simulink model "kinematic_model_pid"  (R2017a)
settings: Solver=ode45  StartTime=0.0  StopTime=5  RelTol=1e-3  EnableMultiTasking=on
InitFcn:
  | S = 1
  | P = 1
  | I = 1
  | D = 1
values from neighbouring files (symbols this model uses):
  Brot = 0    [param_2224.m]
  Bwheel = 0    [param_2224.m]
  Dist_wheels = 0.12    [param_2224.m]
  Jrot = 2.7e-7    (= 2.7e-07)    [param_2224.m]
  Jwheel = 4.013e-6    (= 4.013e-06)    [param_2224.m]
  Ke = 1.115e-3*60/(2*pi)    (= 0.0106474656928)    [param_2224.m]
  Km = 11.12e-3    (= 0.01112)    [param_2224.m]
  L = 130e-6    (= 0.00013)    [param_2224.m]
  n = 8    [param_2224.m]
  R = 8.71    [param_2224.m]
  rads2mps = Rwheel    (= 0.0325)    [param_2224.m]
  rads2rpm = 60/(2*pi)    (= 9.54929658551)    [param_2224.m]
  ro = 0.9    [param_2224.m]
libraries: simulink x11
settings Model: Creator=void  LastModifiedBy=johne
settings DataIOCC: LimitDataPoints=on  SaveFormat=Array  SignalLoggingSaveFormat=ModelDataLogs
settings OptimizationCC: ExpressionDepthLimit=2147483647  InitFltsAndDblsToZero=on  LifeSpan=inf
settings DebuggingCC: SaveWithParameterizedLinksMsg=none  UnderspecifiedInitializationDetection=Classic  MergeDetectMultiDrivingBlocksExec=none  SignalResolutionControl=TryResolveAllWithWarning  SolverPrmCheckMsg=warning  MultiTaskDSMMsg=warning  MultiTaskCondExecSysMsg=none  FcnCallInpInsideContextMsg=warning  StateNameClashWarn=warning  SFUnexpectedBacktrackingDiag=warning  SFNoUnconditionalDefaultTransitionDiag=warning  SFExecutionAtInitializationDiag=none
settings HardwareCC: ProdBitPerPointer=32  ProdBitPerSizeT=32  ProdBitPerPtrDiffT=32  ProdLargestAtomicFloat=None  ProdIntDivRoundTo=Undefined  ProdEndianess=Unspecified  ProdWordSize=32  ProdHWDeviceType=32-bit Generic
settings ModelReferenceCC: PropagateSignalLabelsOutOfModel=off
settings GRTTargetCC: TargetFcnLib=ansi_tfl_tmw.mat  TargetLangStandard=C89/C90 (ANSI)  GeneratePreprocessorConditionals=Disable all  CombineOutputUpdateFcns=off  GRTInterface=on
settings ConfigComp: CovMetricSettings=dw  CovHtmlReporting=on  CovSaveCumulativeToWorkspaceVar=on  CovSaveSingleToWorkspaceVar=on  CovExternalEMLEnable=off

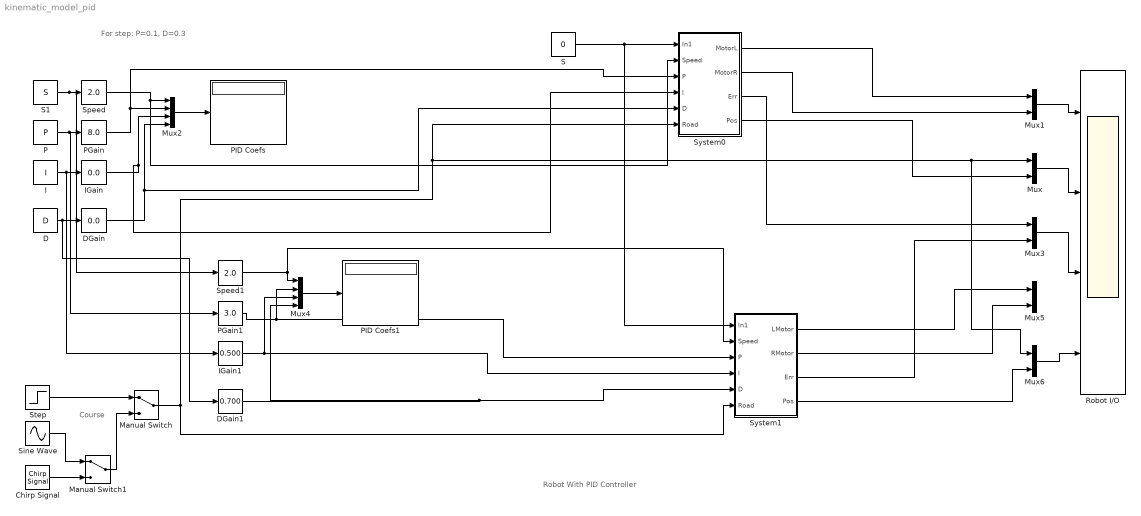
== system kinematic_model_pid ==
  note: For step: P=0.1, D=0.3
  note: Course
  note: Robot With PID Controller
  Chirp Signal : simulink/Sources/Chirp Signal  f1=0.1  T=100  f2=1
  D : Constant  Value=D
  DGain : simulink/Math Operations/Slider Gain  gain=0.0  low=0  high=1
  DGain1 : simulink/Math Operations/Slider Gain  gain=0.700  low=0  high=1
  I : Constant  Value=I
  IGain : simulink/Math Operations/Slider Gain  gain=0.0  low=0  high=1
  IGain1 : simulink/Math Operations/Slider Gain  gain=0.500  low=0  high=1
  Manual Switch : ManualSwitch
  Manual Switch1 : ManualSwitch
  Mux{,1,3,5..6} (5 alike) : Mux  Inputs=2
  Mux2 : Mux
  Mux4 : Mux
  P : Constant  Value=P
  PGain : simulink/Math Operations/Slider Gain  gain=8.0  low=0  high=10
  PGain1 : simulink/Math Operations/Slider Gain  gain=3.0  low=0  high=10
  PID Coefs : Display
  PID Coefs1 : Display
  Robot I/O : Scope  NumInputPorts=4
  S : Constant  Value=0
  S1 : Constant  Value=S
  Sine Wave : Sin  Amplitude=.4  Frequency=2  SampleTime=0
  Speed : simulink/Math Operations/Slider Gain  gain=2.0  low=0  high=10
  Speed1 : simulink/Math Operations/Slider Gain  gain=2.0  low=0  high=10
  Step : Step  After=.5  SampleTime=0
  System0 : Subsystem
  System1 : Subsystem
  wires:
  Speed/1 -> System0/2(Speed), Mux2/1
  Step/1 -> Manual Switch/1
  Manual Switch/1 -> System1/6(Road), System0/6(Road), Mux6/1, Mux/1
  Mux/1 -> Robot I/O/2
  Mux1/1 -> Robot I/O/1
  P/1 -> PGain1/1, PGain/1
  Mux2/1 -> PID Coefs/1
  I/1 -> IGain1/1, IGain/1
  D/1 -> DGain1/1, DGain/1
  Chirp Signal/1 -> Manual Switch1/2
  Manual Switch1/1 -> Manual Switch/2
  Sine Wave/1 -> Manual Switch1/1
  S1/1 -> Speed1/1, Speed/1
  PGain/1 -> System0/3(P), Mux2/2
  IGain/1 -> System0/4(I), Mux2/3
  DGain/1 -> System0/5(D), Mux2/4
  System0/1(MotorL) -> Mux1/1
  System0/2(MotorR) -> Mux1/2
  System0/4(Pos) -> Mux/2
  System0/3(Err) -> Mux3/1
  Mux3/1 -> Robot I/O/3
  System1/3(Err) -> Mux3/2
  Speed1/1 -> System1/2(Speed), Mux4/1
  Mux4/1 -> PID Coefs1/1
  PGain1/1 -> System1/3(P), Mux4/2
  IGain1/1 -> System1/4(I), Mux4/3
  DGain1/1 -> System1/5(D), Mux4/4
  Mux6/1 -> Robot I/O/4
  System1/1(LMotor) -> Mux5/1
  System1/2(RMotor) -> Mux5/2
  System1/4(Pos) -> Mux6/2
  S/1 -> System1/1(In1), System0/1(In1)

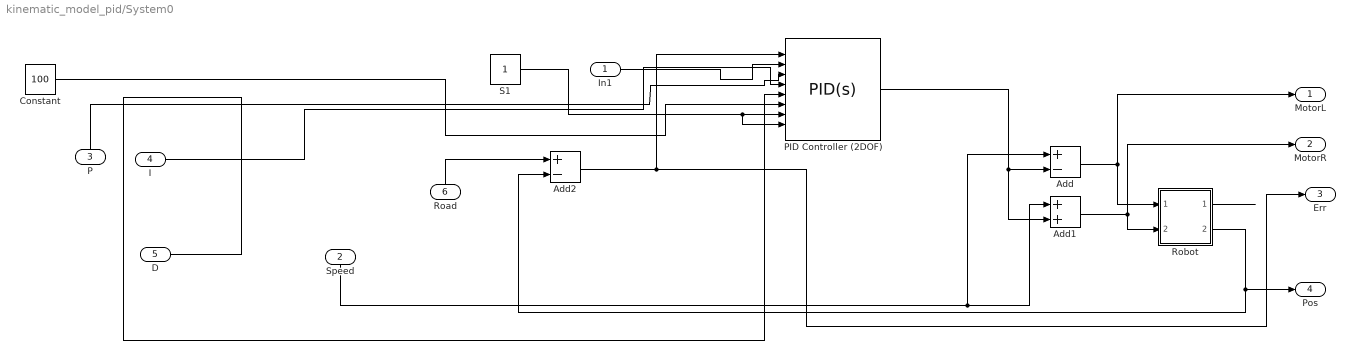
== system kinematic_model_pid/System0 ==
  In1 : Inport
  Speed : Inport  Port=2
  P : Inport  Port=3
  I : Inport  Port=4
  D : Inport  Port=5
  Road : Inport  Port=6
  Add : Sum  Inputs=+-
  Add1 : Sum
  Add2 : Sum  Inputs=+-
  Constant : Constant  Value=100
  PID Controller (2DOF) : simulink/Continuous/PID Controller (2DOF)  Controller=PID  TimeDomain=Continuous-time  SampleTime=-1  IntegratorMethod=Forward Euler  FilterMethod=Forward Euler  Form=Parallel  UseFilter=on  ControllerParametersSource=external  P=1  I=1  D=0  N=100  b=1  c=1  InitialConditionSource=internal  InitialConditionForIntegrator=0  InitialConditionForFilter=0  ExternalReset=none  LimitOutput=off  UpperSaturationLimit=inf  LowerSaturationLimit=-inf  LinearizeAsGain=on  AntiWindupMode=none  Kb=1  TrackingMode=off  Kt=1  PParamMin=[]  PParamMax=[]  IParamMin=[]  IParamMax=[]  DParamMin=[]  DParamMax=[]  NParamMin=[]  NParamMax=[]  bParamMin=[]  bParamMax=[]  cParamMin=[]  cParamMax=[]  KbParamMin=[]  KbParamMax=[]  KtParamMin=[]  KtParamMax=[]  POutMin=[]  POutMax=[]  IOutMin=[]  IOutMax=[]  DOutMin=[]  DOutMax=[]  NOutMin=[]  NOutMax=[]  bOutMin=[]  bOutMax=[]  cOutMin=[]  cOutMax=[]  KbOutMin=[]  KbOutMax=[]  KtOutMin=[]  KtOutMax=[]  IntegratorOutMin=[]  IntegratorOutMax=[]  FilterOutMin=[]  FilterOutMax=[]  SumOutMin=[]  SumOutMax=[]  Sum1OutMin=[]  Sum1OutMax=[]  Sum2OutMin=[]  Sum2OutMax=[]  Sum3OutMin=[]  Sum3OutMax=[]  SumI1OutMin=[]  SumI1OutMax=[]  SumI2OutMin=[]  SumI2OutMax=[]  SumI3OutMin=[]  SumI3OutMax=[]  SumDOutMin=[]  SumDOutMax=[]  SaturationOutMin=[]  SaturationOutMax=[]  IntegratorContinuousStateAttributes=''  IntegratorStateMustResolveToSignalObject=off  IntegratorRTWStateStorageClass=Auto  FilterContinuousStateAttributes=''  FilterStateMustResolveToSignalObject=off  FilterRTWStateStorageClass=Auto  DifferentiatorICPrevScaledInput=0  DifferentiatorOutMin=[]  DifferentiatorOutMax=[]  InitialConditionSetting=State (most efficient)
  Robot : Subsystem
  S1 : Constant
  MotorL : Outport
  MotorR : Outport  Port=2
  Err : Outport  Port=3
  Pos : Outport  Port=4
  wires:
  P/1 -> PID Controller (2DOF)/3
  D/1 -> PID Controller (2DOF)/5
  Road/1 -> Add2/1
  I/1 -> PID Controller (2DOF)/4
  Speed/1 -> Add1/1, Add/1
  In1/1 -> PID Controller (2DOF)/2
  Robot/1(PosX) -> ?
  Add/1 -> MotorL/1, Robot/1(VoltL)
  Add1/1 -> MotorR/1, Robot/2(VoltR)
  Robot/2(PosY) -> Pos/1, Add2/2
  PID Controller (2DOF)/1 -> Add1/2, Add/2
  Add2/1 -> Err/1, PID Controller (2DOF)/1
  S1/1 -> PID Controller (2DOF)/8, PID Controller (2DOF)/7
  Constant/1 -> PID Controller (2DOF)/6

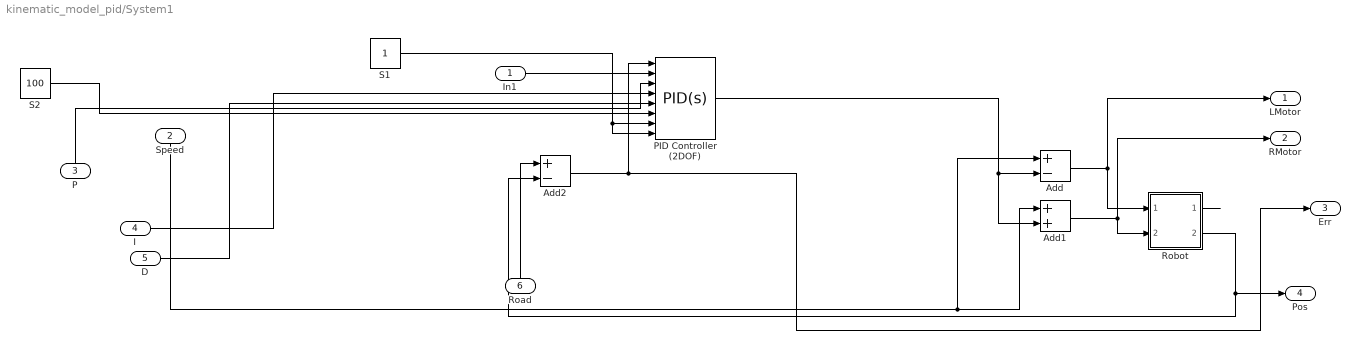
== system kinematic_model_pid/System1 ==
  In1 : Inport
  Speed : Inport  Port=2
  P : Inport  Port=3
  I : Inport  Port=4
  D : Inport  Port=5
  Road : Inport  Port=6
  Add : Sum  Inputs=+-
  Add1 : Sum
  Add2 : Sum  Inputs=+-
  PID Controller (2DOF) : simulink/Continuous/PID Controller (2DOF)  Controller=PID  TimeDomain=Continuous-time  SampleTime=-1  IntegratorMethod=Forward Euler  FilterMethod=Forward Euler  Form=Parallel  UseFilter=on  ControllerParametersSource=external  P=1  I=1  D=0  N=100  b=1  c=1  InitialConditionSource=internal  InitialConditionForIntegrator=0  InitialConditionForFilter=0  ExternalReset=none  LimitOutput=off  UpperSaturationLimit=inf  LowerSaturationLimit=-inf  LinearizeAsGain=on  AntiWindupMode=none  Kb=1  TrackingMode=off  Kt=1  PParamMin=[]  PParamMax=[]  IParamMin=[]  IParamMax=[]  DParamMin=[]  DParamMax=[]  NParamMin=[]  NParamMax=[]  bParamMin=[]  bParamMax=[]  cParamMin=[]  cParamMax=[]  KbParamMin=[]  KbParamMax=[]  KtParamMin=[]  KtParamMax=[]  POutMin=[]  POutMax=[]  IOutMin=[]  IOutMax=[]  DOutMin=[]  DOutMax=[]  NOutMin=[]  NOutMax=[]  bOutMin=[]  bOutMax=[]  cOutMin=[]  cOutMax=[]  KbOutMin=[]  KbOutMax=[]  KtOutMin=[]  KtOutMax=[]  IntegratorOutMin=[]  IntegratorOutMax=[]  FilterOutMin=[]  FilterOutMax=[]  SumOutMin=[]  SumOutMax=[]  Sum1OutMin=[]  Sum1OutMax=[]  Sum2OutMin=[]  Sum2OutMax=[]  Sum3OutMin=[]  Sum3OutMax=[]  SumI1OutMin=[]  SumI1OutMax=[]  SumI2OutMin=[]  SumI2OutMax=[]  SumI3OutMin=[]  SumI3OutMax=[]  SumDOutMin=[]  SumDOutMax=[]  SaturationOutMin=[]  SaturationOutMax=[]  IntegratorContinuousStateAttributes=''  IntegratorStateMustResolveToSignalObject=off  IntegratorRTWStateStorageClass=Auto  FilterContinuousStateAttributes=''  FilterStateMustResolveToSignalObject=off  FilterRTWStateStorageClass=Auto  DifferentiatorICPrevScaledInput=0  DifferentiatorOutMin=[]  DifferentiatorOutMax=[]  InitialConditionSetting=State (most efficient)
  Robot : Subsystem
  S1 : Constant
  S2 : Constant  Value=100
  LMotor : Outport
  RMotor : Outport  Port=2
  Err : Outport  Port=3
  Pos : Outport  Port=4
  wires:
  P/1 -> PID Controller (2DOF)/3
  D/1 -> PID Controller (2DOF)/5
  Road/1 -> Add2/1
  I/1 -> PID Controller (2DOF)/4
  Speed/1 -> Add1/1, Add/1
  In1/1 -> PID Controller (2DOF)/2
  Robot/1(PosX) -> ?
  Add/1 -> LMotor/1, Robot/1(VoltL)
  Add1/1 -> RMotor/1, Robot/2(VoltR)
  Robot/2(PosY) -> Pos/1, Add2/2
  PID Controller (2DOF)/1 -> Add1/2, Add/2
  Add2/1 -> Err/1, PID Controller (2DOF)/1
  S1/1 -> PID Controller (2DOF)/8, PID Controller (2DOF)/7
  S2/1 -> PID Controller (2DOF)/6

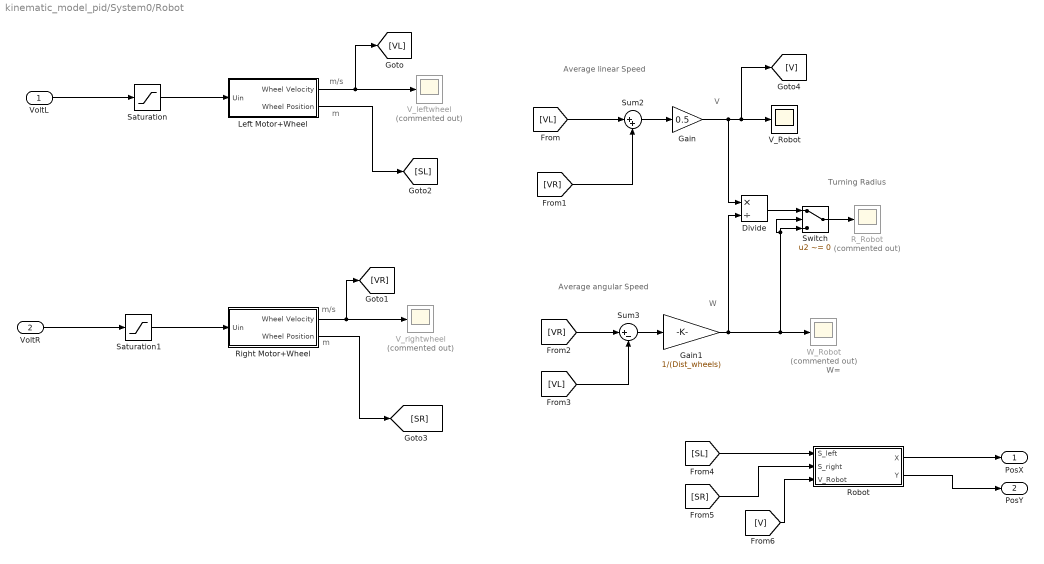
== system kinematic_model_pid/System0/Robot ==
  note: V
  note: W
  note: Average linear Speed
  note: Average angular Speed
  note: Turning Radius
  note: m/s
  note: m
  note: m/s
  note: m
  note: W=
  VoltL : Inport
  VoltR : Inport  Port=2
  Divide : Product  Inputs=*/  SaturateOnIntegerOverflow=on
  Gain : Gain  Gain=0.5
  Gain1 : Gain  Gain=1/(Dist_wheels)
  Left Motor+Wheel : Subsystem
  R_Robot : Scope  Commented=on
  Right Motor+Wheel : Subsystem
  Robot : Subsystem
  Saturation : Saturate  UpperLimit=11.1  LowerLimit=-11.1
  Saturation1 : Saturate  UpperLimit=11.1  LowerLimit=-11.1
  Sum2 : Sum  Inputs=|++
  Sum3 : Sum  Inputs=|+-
  Switch : Switch  Criteria=u2 ~= 0
  V_Robot : Scope
  V_leftwheel : Scope  Commented=on
  V_rightwheel : Scope  Commented=on
  W_Robot : Scope  Commented=on
  PosX : Outport
  PosY : Outport  Port=2
  wires:
  Left Motor+Wheel/1(Wheel Velocity) -> [VL], V_leftwheel/1
  Saturation/1 -> Left Motor+Wheel/1(Uin)
  VoltL/1 -> Saturation/1
  Right Motor+Wheel/1(Wheel Velocity) -> V_rightwheel/1, [VR]
  Saturation1/1 -> Right Motor+Wheel/1(Uin)
  VoltR/1 -> Saturation1/1
  Sum2/1 -> Gain/1
  Gain/1 -> Divide/1, V_Robot/1, [V]
  [VL] -> Sum2/1
  [VR] -> Sum2/2
  Sum3/1 -> Gain1/1
  Gain1/1 -> Divide/2, W_Robot/1, Switch/2, Switch/3
  [VR] -> Sum3/1
  [VL] -> Sum3/2
  Divide/1 -> Switch/1
  Switch/1 -> R_Robot/1
  Right Motor+Wheel/2(Wheel Position) -> [SR]
  Left Motor+Wheel/2(Wheel Position) -> [SL]
  Robot/1(X) -> PosX/1
  Robot/2(Y) -> PosY/1
  [SR] -> Robot/2(S_right)
  [V] -> Robot/3(V_Robot)
  [SL] -> Robot/1(S_left)

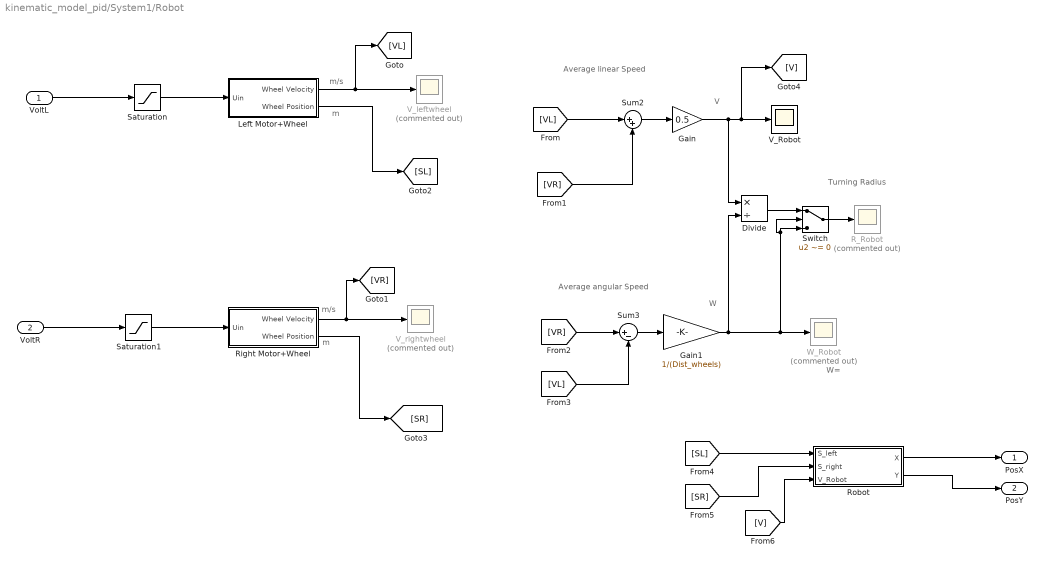
== system kinematic_model_pid/System1/Robot ==
  note: V
  note: W
  note: Average linear Speed
  note: Average angular Speed
  note: Turning Radius
  note: m/s
  note: m
  note: m/s
  note: m
  note: W=
  VoltL : Inport
  VoltR : Inport  Port=2
  Divide : Product  Inputs=*/  SaturateOnIntegerOverflow=on
  Gain : Gain  Gain=0.5
  Gain1 : Gain  Gain=1/(Dist_wheels)
  Left Motor+Wheel : Subsystem
  R_Robot : Scope  Commented=on
  Right Motor+Wheel : Subsystem
  Robot : Subsystem
  Saturation : Saturate  UpperLimit=11.1  LowerLimit=-11.1
  Saturation1 : Saturate  UpperLimit=11.1  LowerLimit=-11.1
  Sum2 : Sum  Inputs=|++
  Sum3 : Sum  Inputs=|+-
  Switch : Switch  Criteria=u2 ~= 0
  V_Robot : Scope
  V_leftwheel : Scope  Commented=on
  V_rightwheel : Scope  Commented=on
  W_Robot : Scope  Commented=on
  PosX : Outport
  PosY : Outport  Port=2
  wires:
  Left Motor+Wheel/1(Wheel Velocity) -> [VL], V_leftwheel/1
  Saturation/1 -> Left Motor+Wheel/1(Uin)
  VoltL/1 -> Saturation/1
  Right Motor+Wheel/1(Wheel Velocity) -> V_rightwheel/1, [VR]
  Saturation1/1 -> Right Motor+Wheel/1(Uin)
  VoltR/1 -> Saturation1/1
  Sum2/1 -> Gain/1
  Gain/1 -> Divide/1, V_Robot/1, [V]
  [VL] -> Sum2/1
  [VR] -> Sum2/2
  Sum3/1 -> Gain1/1
  Gain1/1 -> Divide/2, W_Robot/1, Switch/2, Switch/3
  [VR] -> Sum3/1
  [VL] -> Sum3/2
  Divide/1 -> Switch/1
  Switch/1 -> R_Robot/1
  Right Motor+Wheel/2(Wheel Position) -> [SR]
  Left Motor+Wheel/2(Wheel Position) -> [SL]
  Robot/1(X) -> PosX/1
  Robot/2(Y) -> PosY/1
  [SR] -> Robot/2(S_right)
  [V] -> Robot/3(V_Robot)
  [SL] -> Robot/1(S_left)

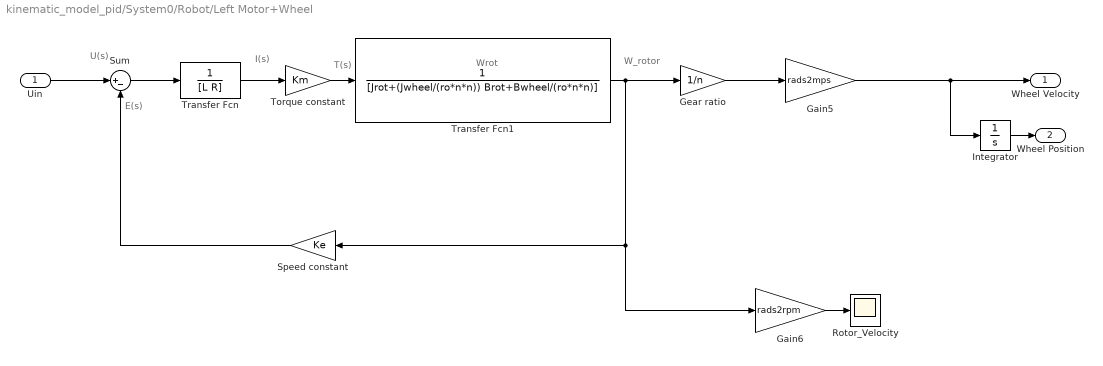
== system kinematic_model_pid/System0/Robot/Left Motor+Wheel ==
  note: I(s)
  note: E(s)
  note: U(s)
  note: T(s)
  note: Wrot
  note: W_rotor
  Uin : Inport
  Gain5 : Gain  Gain=rads2mps
  Gain6 : Gain  Gain=rads2rpm
  Gear ratio : Gain  Gain=1/n
  Integrator : Integrator
  Rotor_Velocity : Scope
  Speed constant : Gain  Gain=Ke
  Sum : Sum  Inputs=|+-
  Torque constant : Gain  Gain=Km
  Transfer Fcn : TransferFcn  Denominator=[L R]
  Transfer Fcn1 : TransferFcn  Denominator=[Jrot+(Jwheel/(ro*n*n)) Brot+Bwheel/(ro*n*n)]
  Wheel Velocity : Outport
  Wheel Position : Outport  Port=2
  wires:
  Sum/1 -> Transfer Fcn/1
  Transfer Fcn/1 -> Torque constant/1
  Torque constant/1 -> Transfer Fcn1/1
  Speed constant/1 -> Sum/2
  Transfer Fcn1/1 -> Gear ratio/1, Speed constant/1, Gain6/1
  Gear ratio/1 -> Gain5/1
  Gain6/1 -> Rotor_Velocity/1
  Uin/1 -> Sum/1
  Gain5/1 -> Wheel Velocity/1, Integrator/1
  Integrator/1 -> Wheel Position/1

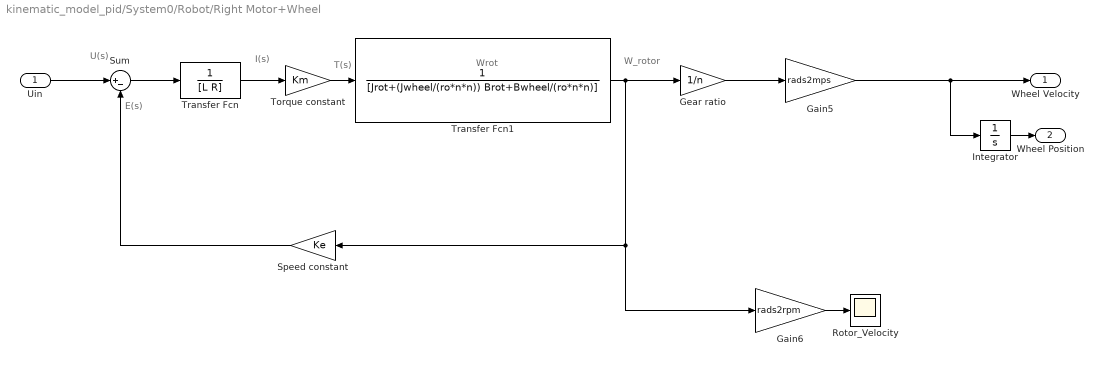
== system kinematic_model_pid/System0/Robot/Right Motor+Wheel ==
  note: I(s)
  note: E(s)
  note: U(s)
  note: T(s)
  note: Wrot
  note: W_rotor
  Uin : Inport
  Gain5 : Gain  Gain=rads2mps
  Gain6 : Gain  Gain=rads2rpm
  Gear ratio : Gain  Gain=1/n
  Integrator : Integrator
  Rotor_Velocity : Scope
  Speed constant : Gain  Gain=Ke
  Sum : Sum  Inputs=|+-
  Torque constant : Gain  Gain=Km
  Transfer Fcn : TransferFcn  Denominator=[L R]
  Transfer Fcn1 : TransferFcn  Denominator=[Jrot+(Jwheel/(ro*n*n)) Brot+Bwheel/(ro*n*n)]
  Wheel Velocity : Outport
  Wheel Position : Outport  Port=2
  wires:
  Sum/1 -> Transfer Fcn/1
  Transfer Fcn/1 -> Torque constant/1
  Torque constant/1 -> Transfer Fcn1/1
  Speed constant/1 -> Sum/2
  Transfer Fcn1/1 -> Gear ratio/1, Speed constant/1, Gain6/1
  Gear ratio/1 -> Gain5/1
  Gain6/1 -> Rotor_Velocity/1
  Uin/1 -> Sum/1
  Gain5/1 -> Wheel Velocity/1, Integrator/1
  Integrator/1 -> Wheel Position/1

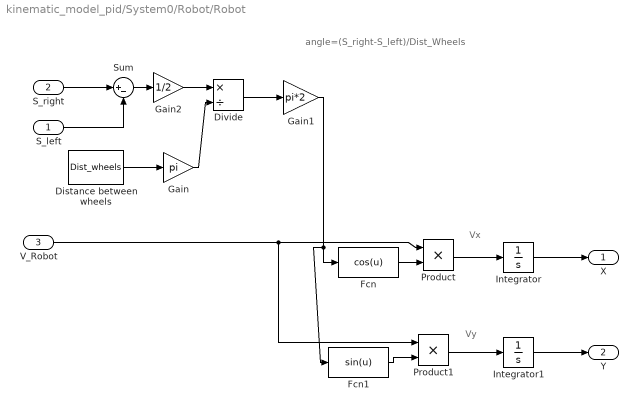
== system kinematic_model_pid/System0/Robot/Robot ==
  note: Vx
  note: Vy
  note: angle=(S_right-S_left)/Dist_Wheels
  S_left : Inport
  S_right : Inport  Port=2
  V_Robot : Inport  Port=3
  Distance between wheels : Constant  Value=Dist_wheels
  Divide : Product  Inputs=*/
  Fcn : Fcn  Expr=cos(u)
  Fcn1 : Fcn  Expr=sin(u)
  Gain : Gain  Gain=pi
  Gain1 : Gain  Gain=pi*2
  Gain2 : Gain  Gain=1/2
  Integrator : Integrator
  Integrator1 : Integrator
  Product : Product  RndMeth=Zero
  Product1 : Product  RndMeth=Zero
  Sum : Sum  Inputs=|+-
  X : Outport
  Y : Outport  Port=2
  wires:
  Distance between wheels/1 -> Gain/1
  Gain/1 -> Divide/2
  Sum/1 -> Gain2/1
  Divide/1 -> Gain1/1
  Gain1/1 -> Fcn/1, Fcn1/1
  Fcn/1 -> Product/2
  Fcn1/1 -> Product1/2
  Product1/1 -> Integrator1/1
  V_Robot/1 -> Product1/1, Product/1
  Product/1 -> Integrator/1
  S_right/1 -> Sum/1
  S_left/1 -> Sum/2
  Gain2/1 -> Divide/1
  Integrator1/1 -> Y/1
  Integrator/1 -> X/1

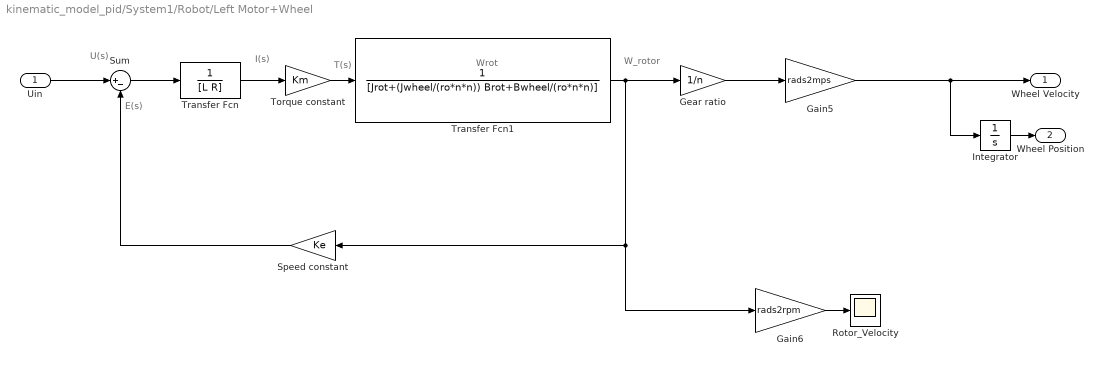
== system kinematic_model_pid/System1/Robot/Left Motor+Wheel ==
  note: I(s)
  note: E(s)
  note: U(s)
  note: T(s)
  note: Wrot
  note: W_rotor
  Uin : Inport
  Gain5 : Gain  Gain=rads2mps
  Gain6 : Gain  Gain=rads2rpm
  Gear ratio : Gain  Gain=1/n
  Integrator : Integrator
  Rotor_Velocity : Scope
  Speed constant : Gain  Gain=Ke
  Sum : Sum  Inputs=|+-
  Torque constant : Gain  Gain=Km
  Transfer Fcn : TransferFcn  Denominator=[L R]
  Transfer Fcn1 : TransferFcn  Denominator=[Jrot+(Jwheel/(ro*n*n)) Brot+Bwheel/(ro*n*n)]
  Wheel Velocity : Outport
  Wheel Position : Outport  Port=2
  wires:
  Sum/1 -> Transfer Fcn/1
  Transfer Fcn/1 -> Torque constant/1
  Torque constant/1 -> Transfer Fcn1/1
  Speed constant/1 -> Sum/2
  Transfer Fcn1/1 -> Gear ratio/1, Speed constant/1, Gain6/1
  Gear ratio/1 -> Gain5/1
  Gain6/1 -> Rotor_Velocity/1
  Uin/1 -> Sum/1
  Gain5/1 -> Wheel Velocity/1, Integrator/1
  Integrator/1 -> Wheel Position/1

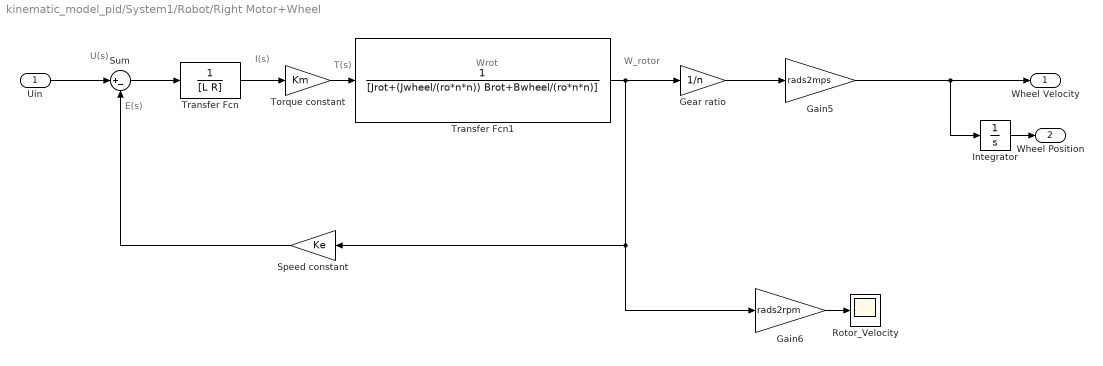
== system kinematic_model_pid/System1/Robot/Right Motor+Wheel ==
  note: I(s)
  note: E(s)
  note: U(s)
  note: T(s)
  note: Wrot
  note: W_rotor
  Uin : Inport
  Gain5 : Gain  Gain=rads2mps
  Gain6 : Gain  Gain=rads2rpm
  Gear ratio : Gain  Gain=1/n
  Integrator : Integrator
  Rotor_Velocity : Scope
  Speed constant : Gain  Gain=Ke
  Sum : Sum  Inputs=|+-
  Torque constant : Gain  Gain=Km
  Transfer Fcn : TransferFcn  Denominator=[L R]
  Transfer Fcn1 : TransferFcn  Denominator=[Jrot+(Jwheel/(ro*n*n)) Brot+Bwheel/(ro*n*n)]
  Wheel Velocity : Outport
  Wheel Position : Outport  Port=2
  wires:
  Sum/1 -> Transfer Fcn/1
  Transfer Fcn/1 -> Torque constant/1
  Torque constant/1 -> Transfer Fcn1/1
  Speed constant/1 -> Sum/2
  Transfer Fcn1/1 -> Gear ratio/1, Speed constant/1, Gain6/1
  Gear ratio/1 -> Gain5/1
  Gain6/1 -> Rotor_Velocity/1
  Uin/1 -> Sum/1
  Gain5/1 -> Wheel Velocity/1, Integrator/1
  Integrator/1 -> Wheel Position/1

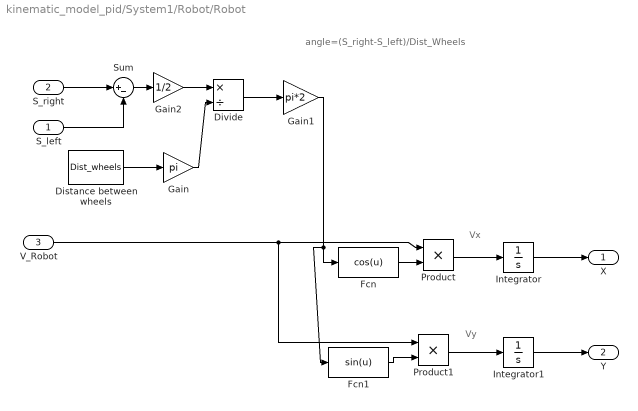
== system kinematic_model_pid/System1/Robot/Robot ==
  note: Vx
  note: Vy
  note: angle=(S_right-S_left)/Dist_Wheels
  S_left : Inport
  S_right : Inport  Port=2
  V_Robot : Inport  Port=3
  Distance between wheels : Constant  Value=Dist_wheels
  Divide : Product  Inputs=*/
  Fcn : Fcn  Expr=cos(u)
  Fcn1 : Fcn  Expr=sin(u)
  Gain : Gain  Gain=pi
  Gain1 : Gain  Gain=pi*2
  Gain2 : Gain  Gain=1/2
  Integrator : Integrator
  Integrator1 : Integrator
  Product : Product  RndMeth=Zero
  Product1 : Product  RndMeth=Zero
  Sum : Sum  Inputs=|+-
  X : Outport
  Y : Outport  Port=2
  wires:
  Distance between wheels/1 -> Gain/1
  Gain/1 -> Divide/2
  Sum/1 -> Gain2/1
  Divide/1 -> Gain1/1
  Gain1/1 -> Fcn/1, Fcn1/1
  Fcn/1 -> Product/2
  Fcn1/1 -> Product1/2
  Product1/1 -> Integrator1/1
  V_Robot/1 -> Product1/1, Product/1
  Product/1 -> Integrator/1
  S_right/1 -> Sum/1
  S_left/1 -> Sum/2
  Gain2/1 -> Divide/1
  Integrator1/1 -> Y/1
  Integrator/1 -> X/1
